simulink model "simpleSimscape"  (R2018a)
settings: Solver=VariableStepAuto  StartTime=0.0  StopTime=10.0  RelTol=1e-3
undefined symbols (not defined in the file): m, s, veh
libraries: fl_lib x9, nesl_utility x5, sdl_lib x3
settings Model: Creator=carca  LastModifiedBy=carca

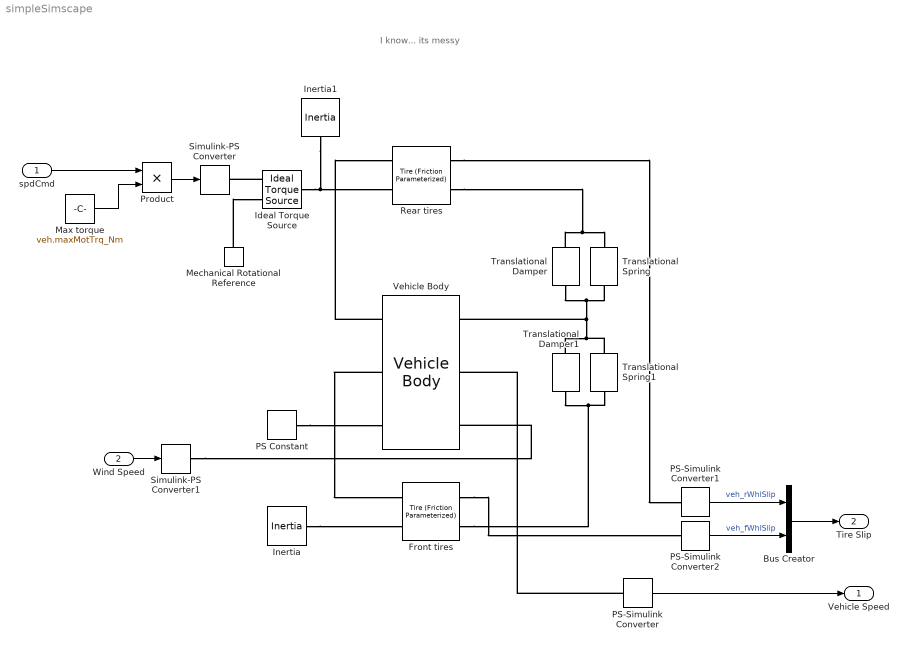
== system simpleSimscape ==
  note: I know... its messy
  spdCmd : Inport
  Wind Speed : Inport  Port=2
  Bus Creator : BusCreator  Inputs=2
  Front tires : sdl_lib/Tires & Vehicles/Tire (Friction Parameterized)  r_tire=veh.whlRad_m m  mu_static=veh.whlStatFric  friction_model=1  mu_kinetic=veh.whlKinFric  slip_vector=[0, .02, .06, .15, .6, 1] rad/s  mu_kinetic_vector=[.89, .88, .8, .75, .7, .7]  interp_method=simscape.enum.interpolation.linear  extrap_method=simscape.enum.extrapolation.linear  model_compliance=0  stiffness=1e6 N/m  damping=1000 N/(m/s)  model_inertia=0  tire_inertia=1 kg*m^2  initial_velocity=0 rad/s  model_resistance=1  resistance_model=1  coeff=veh.rollRstnce  p_tire=250e3 Pa  alpha=-0.003  beta=0.97  coeff_a=84e-4  coeff_b=6.2e-4 s/m  coeff_c=1.6e-4 s^2/m^2  v_thr=0.001 m/s  v_tol=0.01 m/s  F_min=10 N  initial_traction_state=0  mu_static_specify=off  mu_static_priority=None  mu_static_nominal_specify=off  mu_static_nominal_unit=1  mu_static_nominal_value=1  mu_kinetic_specify=off  mu_kinetic_priority=None  mu_kinetic_nominal_specify=off  mu_kinetic_nominal_unit=1  mu_kinetic_nominal_value=1
      settings: SourceProductName=Simscape Driveline  SourceProductBaseCode=LD
  Ideal Torque Source : fl_lib/Mechanical/Mechanical Sources/Ideal Torque Source
  Inertia : fl_lib/Mechanical/Rotational Elements/Inertia  inertia=veh.frWhlInertia_kgms2 kg*m^2  w_specify=off  w_priority=High  w=0 rad/s  w_nominal_specify=off  w_nominal_unit=rad/s  w_nominal_value=1  t_specify=off  t_priority=None  t=0 N*m  t_nominal_specify=off  t_nominal_unit=N*m  t_nominal_value=1
  Inertia1 : fl_lib/Mechanical/Rotational Elements/Inertia  inertia=veh.frWhlInertia_kgms2 kg*m^2  w_specify=off  w_priority=High  w=0 rad/s  w_nominal_specify=off  w_nominal_unit=rad/s  w_nominal_value=1  t_specify=off  t_priority=None  t=0 N*m  t_nominal_specify=off  t_nominal_unit=N*m  t_nominal_value=1
  Max torque : Constant  Value=veh.maxMotTrq_Nm
  Mechanical Rotational Reference : fl_lib/Mechanical/Rotational Elements/Mechanical Rotational Reference
  PS Constant : fl_lib/Physical Signals/Sources/PS Constant  constant=0
  PS-Simulink Converter : nesl_utility/PS-Simulink Converter  PhysicalDomain=network_engine_domain  SubClassName=ps_output  LeftPortType=input  RightPortType=output  PseudoPeriodic=off  Frequencies=[]  Unit=1  AffineConversion=off
  PS-Simulink Converter1 : nesl_utility/PS-Simulink Converter  PhysicalDomain=network_engine_domain  SubClassName=ps_output  LeftPortType=input  RightPortType=output  PseudoPeriodic=off  Frequencies=[]  Unit=1  AffineConversion=off
  PS-Simulink Converter2 : nesl_utility/PS-Simulink Converter  PhysicalDomain=network_engine_domain  SubClassName=ps_output  LeftPortType=input  RightPortType=output  PseudoPeriodic=off  Frequencies=[]  Unit=1  AffineConversion=off
  Product : Product
  Rear tires : sdl_lib/Tires & Vehicles/Tire (Friction Parameterized)  r_tire=veh.whlRad_m m  mu_static=veh.whlStatFric  friction_model=1  mu_kinetic=veh.whlKinFric  slip_vector=[0, .02, .06, .15, .6, 1] rad/s  mu_kinetic_vector=[.89, .88, .8, .75, .7, .7]  interp_method=simscape.enum.interpolation.linear  extrap_method=simscape.enum.extrapolation.linear  model_compliance=0  stiffness=1e6 N/m  damping=1000 N/(m/s)  model_inertia=0  tire_inertia=1 kg*m^2  initial_velocity=0 rad/s  model_resistance=1  resistance_model=1  coeff=veh.whlRollRstnce  p_tire=250e3 Pa  alpha=-0.003  beta=0.97  coeff_a=84e-4  coeff_b=6.2e-4 s/m  coeff_c=1.6e-4 s^2/m^2  v_thr=0.001 m/s  v_tol=0.01 m/s  F_min=10 N  initial_traction_state=0  mu_static_specify=off  mu_static_priority=None  mu_static_nominal_specify=off  mu_static_nominal_unit=1  mu_static_nominal_value=1  mu_kinetic_specify=off  mu_kinetic_priority=None  mu_kinetic_nominal_specify=off  mu_kinetic_nominal_unit=1  mu_kinetic_nominal_value=1
      settings: SourceProductName=Simscape Driveline  SourceProductBaseCode=LD
  Simulink-PS Converter : nesl_utility/Simulink-PS Converter  PhysicalDomain=network_engine_domain  SubClassName=ps_input  LeftPortType=input  RightPortType=output  PseudoPeriodic=off  Frequencies=[]  NoiseDistribution=none  NoiseParameters=[]  Unit=1  AffineConversion=off  FilteringAndDerivatives=provide  SimscapeFilterOrder=1  InputFilterTimeConstant=0.001  UdotUserProvided=0
  Simulink-PS Converter1 : nesl_utility/Simulink-PS Converter  PhysicalDomain=network_engine_domain  SubClassName=ps_input  LeftPortType=input  RightPortType=output  PseudoPeriodic=off  Frequencies=[]  NoiseDistribution=none  NoiseParameters=[]  Unit=1  AffineConversion=off  FilteringAndDerivatives=provide  SimscapeFilterOrder=1  InputFilterTimeConstant=0.001  UdotUserProvided=0
  Translational Damper : fl_lib/Mechanical/Translational Elements/Translational Damper  D=veh.axleDamp_N-m-s N/(m/s)  v_specify=off  v_priority=None  v=0 m/s  v_nominal_specify=off  v_nominal_unit=m/s  v_nominal_value=1  f_specify=off  f_priority=None  f=0 N  f_nominal_specify=off  f_nominal_unit=N  f_nominal_value=1
  Translational Damper1 : fl_lib/Mechanical/Translational Elements/Translational Damper  D=veh.axleDamp_N-m-s N/(m/s)  v_specify=off  v_priority=None  v=0 m/s  v_nominal_specify=off  v_nominal_unit=m/s  v_nominal_value=1  f_specify=off  f_priority=None  f=0 N  f_nominal_specify=off  f_nominal_unit=N  f_nominal_value=1
  Translational Spring : fl_lib/Mechanical/Translational Elements/Translational Spring  spr_rate=veh.axlStiffness_N-m N/m  v_specify=off  v_priority=None  v=0 m/s  v_nominal_specify=off  v_nominal_unit=m/s  v_nominal_value=1  f_specify=off  f_priority=None  f=0 N  f_nominal_specify=off  f_nominal_unit=N  f_nominal_value=1  x_specify=off  x_priority=High  x=0 m  x_nominal_specify=off  x_nominal_unit=m  x_nominal_value=1
  Translational Spring1 : fl_lib/Mechanical/Translational Elements/Translational Spring  spr_rate=veh.axlStiffness_N-m N/m  v_specify=off  v_priority=None  v=0 m/s  v_nominal_specify=off  v_nominal_unit=m/s  v_nominal_value=1  f_specify=off  f_priority=None  f=0 N  f_nominal_specify=off  f_nominal_unit=N  f_nominal_value=1  x_specify=off  x_priority=High  x=0 m  x_nominal_specify=off  x_nominal_unit=m  x_nominal_value=1
  Vehicle Body : sdl_lib/Tires & Vehicles/Vehicle Body  mass=veh.mass_kg kg  n_w=2  x_f=1.4 m  x_r=1.6 m  y_c=0.5 m  model_pitch=0  inertia=4000 kg*m^2  suspension_model=1  k_f=1e4 N/m  b_f=1e4 N/(m/s)  k_r=1e4 N/m  b_r=1e4 N/(m/s)  k_f_TLU=[-2000, -1000, 0, 1000, 2000] N  x_f_TLU=[-.4, -.2, 0, .2, .4] m  b_f_TLU=[-200, -100, 0, 100, 200] N  v_f_TLU=[-4, -2, 0, 2, 4] m/s  k_r_TLU=[-2000, -1000, 0, 1000, 2000] N  x_r_TLU=[-.4, -.2, 0, .2, .4] m  b_r_TLU=[-200, -100, 0, 100, 200] N  v_r_TLU=[-4, -2, 0, 2, 4] m/s  interp_method=simscape.enum.interpolation.linear  extrap_method=simscape.enum.extrapolation.linear  model_hardstop=0  upper_bound_f=.25 m  lower_bound_f=-.25 m  stop_k_f=1e6 N/m  stop_b_f=150 N/(m/s)  upper_bound_r=.25 m  lower_bound_r=-.25 m  stop_k_r=1e6 N/m  stop_b_r=150 N/(m/s)  initial_pitch=0 rad  initial_pitch_rate=0 rad/s  g=9.81 m/s^2  liftoff_warning=0  area=3 m^2  Cd=0.4  rho=1.18 kg/m^3  v_specify=off  v_priority=High  v=0 m/s  v_nominal_specify=off  v_nominal_unit=m/s  v_nominal_value=1
      settings: SourceProductName=Simscape Driveline
  Vehicle Speed : Outport
  Tire Slip : Outport  Port=2
  wires:
  PS-Simulink Converter/1 -> Vehicle Speed/1
  PS-Simulink Converter1/1 -> Bus Creator/1  "veh_rWhlSlip"
  PS-Simulink Converter2/1 -> Bus Creator/2  "veh_fWhlSlip"
  Bus Creator/1 -> Tire Slip/1
  Wind Speed/1 -> Simulink-PS Converter1/1
  spdCmd/1 -> Product/1
  Max torque/1 -> Product/2
  Product/1 -> Simulink-PS Converter/1
  connections:
  Vehicle Body/RConn1 -- Rear tires/LConn1
  Ideal Torque Source/LConn1 -- Inertia1/LConn1 -- Rear tires/LConn2
  Ideal Torque Source/RConn1 -- Simulink-PS Converter/RConn1
  Mechanical Rotational Reference/LConn1 -- Ideal Torque Source/RConn2
  Translational Damper/LConn1 -- Rear tires/RConn2 -- Translational Spring/LConn1
  Translational Damper/RConn1 -- Translational Spring1/RConn1 -- Translational Damper1/RConn1 -- Vehicle Body/LConn1 -- Translational Spring/RConn1
  Front tires/RConn2 -- Translational Spring1/LConn1 -- Translational Damper1/LConn1
  Vehicle Body/RConn2 -- Front tires/LConn1
  PS Constant/RConn1 -- Vehicle Body/RConn3
  Inertia/LConn1 -- Front tires/LConn2
  PS-Simulink Converter/LConn1 -- Vehicle Body/LConn2
  Rear tires/RConn1 -- PS-Simulink Converter1/LConn1
  Front tires/RConn1 -- PS-Simulink Converter2/LConn1
  Simulink-PS Converter1/RConn1 -- Vehicle Body/LConn3
